simulink model "sf_slscheduler"  (Simulink 7.6)
settings: Solver=FixedStepDiscrete  StartTime=0.0  StopTime=10.0  FixedStep=0.01  RelTol=1e-3
settings Model: Creator=The MathWorks Inc.
settings DebuggingCC: StrictBusMsg=Warning
settings SFSimCC: SimParseCustomCode=off

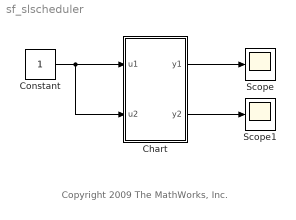
== system sf_slscheduler ==
  note: Copyright 2009 The MathWorks, Inc.
  Chart : Stateflow chart  TreatAsAtomicUnit=on
  Constant : Constant
  Scope : Scope
      settings: YMin=0  YMax=350
  Scope1 : Scope
      settings: YMin=0  YMax=350
  wires:
  Constant/1 -> Chart/1(u1), Chart/2(u2)
  Chart/1(y1) -> Scope/1
  Chart/2(y2) -> Scope1/1

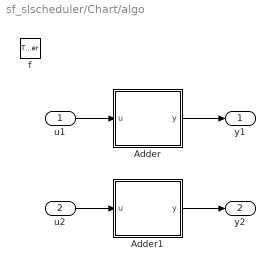
== system sf_slscheduler/Chart/algo ==
  u1 : Inport
  u2 : Inport  Port=2
  f : TriggerPort  TriggerType=function-call
      settings: CopyFcn=set_param(gcbh,'PreDeleteFcn','')  PreDeleteFcn=Stateflow.SLINSF.SimulinkMan.unsafePredeleteFcn
  Adder : Subsystem
  Adder1 : Subsystem
  y1 : Outport
  y2 : Outport  Port=2
  wires:
  u1/1 -> Adder/1(u)
  Adder/1(y) -> y1/1
  u2/1 -> Adder1/1(u)
  Adder1/1(y) -> y2/1

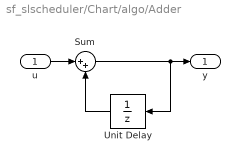
== system sf_slscheduler/Chart/algo/Adder ==
  u : Inport
  Sum : Sum  Inputs=|++
  Unit Delay : UnitDelay  SampleTime=-1
  y : Outport
  wires:
  Sum/1 -> Unit Delay/1, y/1
  Unit Delay/1 -> Sum/2
  u/1 -> Sum/1

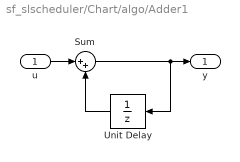
== system sf_slscheduler/Chart/algo/Adder1 ==
  u : Inport
  Sum : Sum  Inputs=|++
  Unit Delay : UnitDelay  SampleTime=-1
  y : Outport
  wires:
  u/1 -> Sum/1
  Unit Delay/1 -> Sum/2
  Sum/1 -> y/1, Unit Delay/1

== stateflow chart Chart ==
  state FAST
    on every(2,tick): [y1,y2] = algo(u1,u2);
  state SLOW
    on every(5,tick): [y1,y2] = algo(u1,u2);
  state [y1,y2] = algo(u1,u2) [function]
  FAST -> SLOW : after(50,tick)
  SLOW -> FAST : after(75,tick)
  (default) -> FAST
  data: u1 function_input double; u2 function_input double; y1 function_output double; y2 function_output double; u1 input double; u2 input double; y1 output double; y2 output double
